simulink model "satellite"  (R2025b)
settings: Solver=VariableStepAuto  StartTime=0.0  StopTime=5  RelTol=1e-3
values from neighbouring files (symbols this model uses):
  A = [0 0 0 1 0 0 ... (first row only)    [Design_Project_Demo_4_5_satellite.m]
  B = [zeros(3,3);eye(3)]    [Design_Project_Demo_4_5_satellite.m]
  F0 = R2I*B'*Pi    [Design_Project_Demo_4_5_satellite.m]
  x0 = [10000; 10000; -10000; 2; 1; 3]    [Design_Project_Demo_4_5_satellite.m]
settings Model: Creator=Zoran Gaijc  LastModifiedBy=gajic

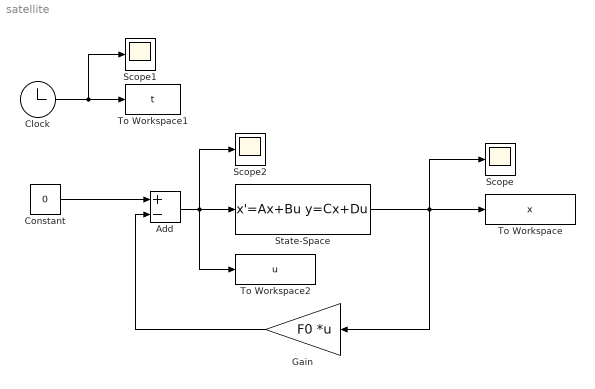
== system satellite ==
  Add : Sum  Inputs=+-
  Clock : Clock
  Constant : Constant  Value=0
  Gain : Gain  Gain=F0  Multiplication=Matrix(K*u)
  Scope : Scope
      settings: ActiveDisplayYMinimum=-1  ActiveDisplayYMaximum=1
  Scope1 : Scope
      settings: ActiveDisplayYMinimum=-0.625  ActiveDisplayYMaximum=5.625
  Scope2 : Scope
      settings: ActiveDisplayYMinimum=-1  ActiveDisplayYMaximum=1  DataLoggingVariableName=ScopeData2
  State-Space : StateSpace  A=A  B=B  C=eye(6)  D=zeros(6,3)  InitialCondition=x0
  To Workspace : ToWorkspace  VariableName=x  SampleTime=-1
  To Workspace1 : ToWorkspace  VariableName=t  SampleTime=-1
  To Workspace2 : ToWorkspace  VariableName=u  SampleTime=-1
  wires:
  Add/1 -> Scope2/1, To Workspace2/1, State-Space/1
  Gain/1 -> Add/2
  State-Space/1 -> Scope/1, To Workspace/1, Gain/1
  Clock/1 -> Scope1/1, To Workspace1/1
  Constant/1 -> Add/1
